simulink model "kurtosis"  (R2012b)
settings: Solver=ode45  StartTime=0.0  StopTime=3171  RelTol=1e-3
libraries: xbsIndex_r4 x3174, casper_library_flow_control x64, casper_library_misc x1, simulink_xsg_bridge x1
(part 6 of 24)

== system kurtosis/kurtosis/kurtosis_acc_bank_6/abs_x_4th_acc ==
  sync : Inport
  b : Inport  Port=2
  Convert : xbsIndex_r4/Convert  gui_display_data_type=Fixed-point  arith_type="Signed  (2's comp)"  n_bits=96  bin_pt=68  float_type=Single  exp_bits=8  fraction_bits=24  quantization=Truncate  overflow=Wrap  en=off  latency=0  dbl_ovrd=off  pipeline=off  block_type=convert
  DSP48E_0 : xbsIndex_r4/DSP48E  use_a=Direct from A Port  use_b=Direct from B Port  reset_preg=off  pattern_from_creg=on  pattern='000000000000'  mask_from_creg=on  pattern_mask='000000000000'  sel_rounding_mask=Select mask  use_op=off  use_creg=on  rst_all=off  en_all=off  use_pcin=off  use_carrycascin=off  use_multsignin=off  use_carryout=on  use_patterndetect=off  use_patternbdetect=off  use_overflow=off  use_underflow=off  use_acout=off  use_bcout=off  use_pcout=off  use_multsignout=off  use_carrycascout=off  pipeline_a=1  pipeline_b=1  pipeline_acout=1  pipeline_bcout=1  pipeline_c=on  pipeline_p=on  pipeline_mult=on  pipeline_opmode=on  pipeline_alumode=on  pipeline_carryin=on  pipeline_carryinsel=on  rst_a=off  rst_b=off  rst_c=off  rst_mult=off  rst_p=off  rst_carry_in=off  rst_alumode=off  rst_ctrl=off  en_a1=off  en_a2=off  en_b1=off  en_b2=off  en_c=off  en_mult=off  en_p=off  en_carry_in=off  en_alumode=off  en_multcarryin=off  en_ctrl=off  use_synth_model=off  addsub_mode=ONE48  xl_useadderonly=off  block_type=dsp48e
  DSP48E_1 : xbsIndex_r4/DSP48E  use_a=Direct from A Port  use_b=Direct from B Port  reset_preg=off  pattern_from_creg=on  pattern='000000000000'  mask_from_creg=on  pattern_mask='000000000000'  sel_rounding_mask=Select mask  use_op=off  use_creg=off  rst_all=off  en_all=off  use_pcin=off  use_carrycascin=off  use_multsignin=off  use_carryout=off  use_patterndetect=off  use_patternbdetect=off  use_overflow=off  use_underflow=off  use_acout=off  use_bcout=off  use_pcout=off  use_multsignout=off  use_carrycascout=off  pipeline_a=2  pipeline_b=2  pipeline_acout=1  pipeline_bcout=1  pipeline_c=on  pipeline_p=on  pipeline_mult=on  pipeline_opmode=on  pipeline_alumode=on  pipeline_carryin=off  pipeline_carryinsel=on  rst_a=off  rst_b=off  rst_c=off  rst_mult=off  rst_p=off  rst_carry_in=off  rst_alumode=off  rst_ctrl=off  en_a1=off  en_a2=off  en_b1=off  en_b2=off  en_c=off  en_mult=off  en_p=off  en_carry_in=off  en_alumode=off  en_multcarryin=off  en_ctrl=off  use_synth_model=off  addsub_mode=ONE48  xl_useadderonly=off  block_type=dsp48e
  DSP48_AB_splitter1 : Subsystem
  DSP48_AB_splitter2_sub : Subsystem
  Delay1 : xbsIndex_r4/Delay  rst=off  infoeditControl=Selection of Reset will increase slice count due to use of real FFs and instead of SRLs  en=off  latency=1  dbl_ovrd=off  reg_retiming=off  block_type=delay
  Mux : xbsIndex_r4/Mux  inputs=2  en=off  latency=0  precision=Full  arith_type=Unsigned  n_bits=16  bin_pt=14  quantization=Truncate  overflow=Wrap  dbl_ovrd=off  block_type=mux
  Mux1 : xbsIndex_r4/Mux  inputs=2  en=off  latency=0  precision=Full  arith_type=Unsigned  n_bits=16  bin_pt=14  quantization=Truncate  overflow=Wrap  dbl_ovrd=off  block_type=mux
  Register : xbsIndex_r4/Register  init=0  rst=off  en=off  dbl_ovrd=off  block_type=register
  Reinterpret : xbsIndex_r4/Reinterpret  force_arith_type=on  arith_type="Signed  (2's comp)"  force_bin_pt=on  bin_pt=0  block_type=reinterpret
  Reinterpret1 : xbsIndex_r4/Reinterpret  force_arith_type=on  arith_type="Signed  (2's comp)"  force_bin_pt=on  bin_pt=0  block_type=reinterpret
  Reinterpret2 : xbsIndex_r4/Reinterpret  force_arith_type=on  arith_type="Signed  (2's comp)"  force_bin_pt=on  bin_pt=68  block_type=reinterpret
  Slice : xbsIndex_r4/Slice  nbits=48  boolean_output=off  mode=Lower Bit Location + Width  bit1=0  base1=MSB of Input  bit0=0  base0=LSB of Input  dbl_ovrd=off  block_type=slice
  Slice2 : xbsIndex_r4/Slice  nbits=48  boolean_output=off  mode=Lower Bit Location + Width  bit1=0  base1=MSB of Input  bit0=48  base0=LSB of Input  dbl_ovrd=off  block_type=slice
  cram : Subsystem
  dsp48e_ctrl_init_xblock94 : Subsystem
  dsp48e_ctrl_init_xblock95 : Subsystem
  opmode_0_rst : xbsIndex_r4/Constant  const=12  gui_display_data_type=Fixed-point  arith_type=Unsigned  n_bits=7  bin_pt=0  preci_type=Single  exp_width=8  frac_width=24  explicit_period=on  period=1  equ=P=C  opselect=C  inp2=PCIN>>17  opr=+  inp1=P  carry=CIN  dbl_ovrd=off  block_type=constant
  opmode_1_rst : xbsIndex_r4/Constant  const=3  gui_display_data_type=Fixed-point  arith_type=Unsigned  n_bits=7  bin_pt=0  preci_type=Single  exp_width=8  frac_width=24  explicit_period=on  period=1  equ=P=C  opselect=C  inp2=PCIN>>17  opr=+  inp1=P  carry=CIN  dbl_ovrd=off  block_type=constant
  zero : xbsIndex_r4/Constant  const=0  gui_display_data_type=Fixed-point  arith_type=Signed (2's comp)  n_bits=48  bin_pt=0  preci_type=Single  exp_width=8  frac_width=24  explicit_period=on  period=1  equ=P=C  opselect=C  inp2=PCIN>>17  opr=+  inp1=P  carry=CIN  dbl_ovrd=off  block_type=constant
  +=b : Outport
  wires:
  sync/1 -> Mux1/1, Mux/1
  Reinterpret1/1 -> Slice2/1, Slice/1  "Reinterpret1_out1"
  dsp48e_ctrl_init_xblock95/4(carryinsel) -> DSP48E_1/6  "dsp48e_ctrl1_out4"
  dsp48e_ctrl_init_xblock95/2(alumode) -> DSP48E_1/4  "dsp48e_ctrl1_out2"
  dsp48e_ctrl_init_xblock95/1(opmode) -> Mux1/2  "dsp48e_ctrl1_out1"
  dsp48e_ctrl_init_xblock94/4(carryinsel) -> DSP48E_0/7  "dsp48e_ctrl0_out4"
  dsp48e_ctrl_init_xblock94/3(carryin) -> DSP48E_0/6  "dsp48e_ctrl0_out3"
  dsp48e_ctrl_init_xblock94/2(alumode) -> DSP48E_0/5  "dsp48e_ctrl0_out2"
  dsp48e_ctrl_init_xblock94/1(opmode) -> Mux/2  "dsp48e_ctrl0_out1"
  DSP48_AB_splitter2_sub/2(B) -> DSP48E_1/2  "DSP48_AB_splitter2_out2"
  DSP48_AB_splitter2_sub/1(A) -> DSP48E_1/1  "DSP48_AB_splitter2_out1"
  Slice2/1 -> DSP48_AB_splitter2_sub/1(A:B)  "Slice2_out1"
  zero/1 -> DSP48_AB_splitter1/1(A:B)  "zero_out1"
  opmode_1_rst/1 -> Mux1/3  "opmode_1_rst_out1"
  opmode_0_rst/1 -> Mux/3  "opmode_0_rst_out1"
  cram/1(Out) -> Reinterpret2/1  "cram_out1"
  Register/1 -> cram/2(In2)  "Register_out1"
  DSP48E_1/1 -> cram/1(In1)  "DSP48E_1_out1"
  Slice/1 -> Reinterpret/1  "Slice_out1"
  Reinterpret2/1 -> +=b/1
  Convert/1 -> Reinterpret1/1  "Convert_out1"
  Reinterpret/1 -> DSP48E_0/3  "Reinterpret_out1"
  DSP48E_0/1 -> Register/1  "DSP48E_0_out1"
  Mux1/1 -> Delay1/1  "Mux1_out1"
  Mux/1 -> DSP48E_0/4  "Mux_out1"
  Delay1/1 -> DSP48E_1/3  "Delay1_out1"
  DSP48_AB_splitter1/2(B) -> DSP48E_0/2  "DSP48_AB_splitter1_out2"
  DSP48_AB_splitter1/1(A) -> DSP48E_0/1  "DSP48_AB_splitter1_out1"
  DSP48E_0/2 -> DSP48E_1/5  "DSP48E_0_out2"
  b/1 -> Convert/1

== system kurtosis/kurtosis/kurtosis_acc_bank_6/abs_x_sq_acc ==
  sync : Inport
  b : Inport  Port=2
  Convert : xbsIndex_r4/Convert  gui_display_data_type=Fixed-point  arith_type="Signed  (2's comp)"  n_bits=96  bin_pt=34  float_type=Single  exp_bits=8  fraction_bits=24  quantization=Truncate  overflow=Wrap  en=off  latency=0  dbl_ovrd=off  pipeline=off  block_type=convert
  DSP48E_0 : xbsIndex_r4/DSP48E  use_a=Direct from A Port  use_b=Direct from B Port  reset_preg=off  pattern_from_creg=on  pattern='000000000000'  mask_from_creg=on  pattern_mask='000000000000'  sel_rounding_mask=Select mask  use_op=off  use_creg=on  rst_all=off  en_all=off  use_pcin=off  use_carrycascin=off  use_multsignin=off  use_carryout=on  use_patterndetect=off  use_patternbdetect=off  use_overflow=off  use_underflow=off  use_acout=off  use_bcout=off  use_pcout=off  use_multsignout=off  use_carrycascout=off  pipeline_a=1  pipeline_b=1  pipeline_acout=1  pipeline_bcout=1  pipeline_c=on  pipeline_p=on  pipeline_mult=on  pipeline_opmode=on  pipeline_alumode=on  pipeline_carryin=on  pipeline_carryinsel=on  rst_a=off  rst_b=off  rst_c=off  rst_mult=off  rst_p=off  rst_carry_in=off  rst_alumode=off  rst_ctrl=off  en_a1=off  en_a2=off  en_b1=off  en_b2=off  en_c=off  en_mult=off  en_p=off  en_carry_in=off  en_alumode=off  en_multcarryin=off  en_ctrl=off  use_synth_model=off  addsub_mode=ONE48  xl_useadderonly=off  block_type=dsp48e
  DSP48E_1 : xbsIndex_r4/DSP48E  use_a=Direct from A Port  use_b=Direct from B Port  reset_preg=off  pattern_from_creg=on  pattern='000000000000'  mask_from_creg=on  pattern_mask='000000000000'  sel_rounding_mask=Select mask  use_op=off  use_creg=off  rst_all=off  en_all=off  use_pcin=off  use_carrycascin=off  use_multsignin=off  use_carryout=off  use_patterndetect=off  use_patternbdetect=off  use_overflow=off  use_underflow=off  use_acout=off  use_bcout=off  use_pcout=off  use_multsignout=off  use_carrycascout=off  pipeline_a=2  pipeline_b=2  pipeline_acout=1  pipeline_bcout=1  pipeline_c=on  pipeline_p=on  pipeline_mult=on  pipeline_opmode=on  pipeline_alumode=on  pipeline_carryin=off  pipeline_carryinsel=on  rst_a=off  rst_b=off  rst_c=off  rst_mult=off  rst_p=off  rst_carry_in=off  rst_alumode=off  rst_ctrl=off  en_a1=off  en_a2=off  en_b1=off  en_b2=off  en_c=off  en_mult=off  en_p=off  en_carry_in=off  en_alumode=off  en_multcarryin=off  en_ctrl=off  use_synth_model=off  addsub_mode=ONE48  xl_useadderonly=off  block_type=dsp48e
  DSP48_AB_splitter1 : Subsystem
  DSP48_AB_splitter2_sub : Subsystem
  Delay1 : xbsIndex_r4/Delay  rst=off  infoeditControl=Selection of Reset will increase slice count due to use of real FFs and instead of SRLs  en=off  latency=1  dbl_ovrd=off  reg_retiming=off  block_type=delay
  Mux : xbsIndex_r4/Mux  inputs=2  en=off  latency=0  precision=Full  arith_type=Unsigned  n_bits=16  bin_pt=14  quantization=Truncate  overflow=Wrap  dbl_ovrd=off  block_type=mux
  Mux1 : xbsIndex_r4/Mux  inputs=2  en=off  latency=0  precision=Full  arith_type=Unsigned  n_bits=16  bin_pt=14  quantization=Truncate  overflow=Wrap  dbl_ovrd=off  block_type=mux
  Register : xbsIndex_r4/Register  init=0  rst=off  en=off  dbl_ovrd=off  block_type=register
  Reinterpret : xbsIndex_r4/Reinterpret  force_arith_type=on  arith_type="Signed  (2's comp)"  force_bin_pt=on  bin_pt=0  block_type=reinterpret
  Reinterpret1 : xbsIndex_r4/Reinterpret  force_arith_type=on  arith_type="Signed  (2's comp)"  force_bin_pt=on  bin_pt=0  block_type=reinterpret
  Reinterpret2 : xbsIndex_r4/Reinterpret  force_arith_type=on  arith_type="Signed  (2's comp)"  force_bin_pt=on  bin_pt=34  block_type=reinterpret
  Slice : xbsIndex_r4/Slice  nbits=48  boolean_output=off  mode=Lower Bit Location + Width  bit1=0  base1=MSB of Input  bit0=0  base0=LSB of Input  dbl_ovrd=off  block_type=slice
  Slice2 : xbsIndex_r4/Slice  nbits=48  boolean_output=off  mode=Lower Bit Location + Width  bit1=0  base1=MSB of Input  bit0=48  base0=LSB of Input  dbl_ovrd=off  block_type=slice
  cram : Subsystem
  dsp48e_ctrl_init_xblock92 : Subsystem
  dsp48e_ctrl_init_xblock93 : Subsystem
  opmode_0_rst : xbsIndex_r4/Constant  const=12  gui_display_data_type=Fixed-point  arith_type=Unsigned  n_bits=7  bin_pt=0  preci_type=Single  exp_width=8  frac_width=24  explicit_period=on  period=1  equ=P=C  opselect=C  inp2=PCIN>>17  opr=+  inp1=P  carry=CIN  dbl_ovrd=off  block_type=constant
  opmode_1_rst : xbsIndex_r4/Constant  const=3  gui_display_data_type=Fixed-point  arith_type=Unsigned  n_bits=7  bin_pt=0  preci_type=Single  exp_width=8  frac_width=24  explicit_period=on  period=1  equ=P=C  opselect=C  inp2=PCIN>>17  opr=+  inp1=P  carry=CIN  dbl_ovrd=off  block_type=constant
  zero : xbsIndex_r4/Constant  const=0  gui_display_data_type=Fixed-point  arith_type=Signed (2's comp)  n_bits=48  bin_pt=0  preci_type=Single  exp_width=8  frac_width=24  explicit_period=on  period=1  equ=P=C  opselect=C  inp2=PCIN>>17  opr=+  inp1=P  carry=CIN  dbl_ovrd=off  block_type=constant
  +=b : Outport
  wires:
  sync/1 -> Mux1/1, Mux/1
  Reinterpret1/1 -> Slice2/1, Slice/1  "Reinterpret1_out1"
  dsp48e_ctrl_init_xblock93/4(carryinsel) -> DSP48E_1/6  "dsp48e_ctrl1_out4"
  dsp48e_ctrl_init_xblock93/2(alumode) -> DSP48E_1/4  "dsp48e_ctrl1_out2"
  dsp48e_ctrl_init_xblock93/1(opmode) -> Mux1/2  "dsp48e_ctrl1_out1"
  dsp48e_ctrl_init_xblock92/4(carryinsel) -> DSP48E_0/7  "dsp48e_ctrl0_out4"
  dsp48e_ctrl_init_xblock92/3(carryin) -> DSP48E_0/6  "dsp48e_ctrl0_out3"
  dsp48e_ctrl_init_xblock92/2(alumode) -> DSP48E_0/5  "dsp48e_ctrl0_out2"
  dsp48e_ctrl_init_xblock92/1(opmode) -> Mux/2  "dsp48e_ctrl0_out1"
  DSP48_AB_splitter2_sub/2(B) -> DSP48E_1/2  "DSP48_AB_splitter2_out2"
  DSP48_AB_splitter2_sub/1(A) -> DSP48E_1/1  "DSP48_AB_splitter2_out1"
  Slice2/1 -> DSP48_AB_splitter2_sub/1(A:B)  "Slice2_out1"
  zero/1 -> DSP48_AB_splitter1/1(A:B)  "zero_out1"
  opmode_1_rst/1 -> Mux1/3  "opmode_1_rst_out1"
  opmode_0_rst/1 -> Mux/3  "opmode_0_rst_out1"
  cram/1(Out) -> Reinterpret2/1  "cram_out1"
  Register/1 -> cram/2(In2)  "Register_out1"
  DSP48E_1/1 -> cram/1(In1)  "DSP48E_1_out1"
  Slice/1 -> Reinterpret/1  "Slice_out1"
  Reinterpret2/1 -> +=b/1
  Convert/1 -> Reinterpret1/1  "Convert_out1"
  Reinterpret/1 -> DSP48E_0/3  "Reinterpret_out1"
  DSP48E_0/1 -> Register/1  "DSP48E_0_out1"
  Mux1/1 -> Delay1/1  "Mux1_out1"
  Mux/1 -> DSP48E_0/4  "Mux_out1"
  Delay1/1 -> DSP48E_1/3  "Delay1_out1"
  DSP48_AB_splitter1/2(B) -> DSP48E_0/2  "DSP48_AB_splitter1_out2"
  DSP48_AB_splitter1/1(A) -> DSP48E_0/1  "DSP48_AB_splitter1_out1"
  DSP48E_0/2 -> DSP48E_1/5  "DSP48E_0_out2"
  b/1 -> Convert/1

== system kurtosis/kurtosis/kurtosis_acc_bank_6/acc_rst ==
  sync : Inport
  Constant5 : xbsIndex_r4/Constant  const=1023  gui_display_data_type=Fixed-point  arith_type=Unsigned  n_bits=11  bin_pt=0  preci_type=Single  exp_width=8  frac_width=24  explicit_period=on  period=1  equ=P=C  opselect=C  inp2=PCIN>>17  opr=+  inp1=P  carry=CIN  dbl_ovrd=off  block_type=constant
  Counter : xbsIndex_r4/Counter  cnt_type=Free Running  cnt_to=Inf  operation=Up  start_count=0  cnt_by_val=1  arith_type=Unsigned  n_bits=10  bin_pt=0  load_pin=off  rst=on  en=off  explicit_period=on  period=1  dbl_ovrd=off  use_behavioral_HDL=off  implementation=Fabric  block_type=counter
  Logical : xbsIndex_r4/Logical  logical_function=OR  inputs=2  en=off  latency=0  precision=Full  arith_type=Unsigned  n_bits=16  bin_pt=0  align_bp=on  dbl_ovrd=off  block_type=logical
  Relational : xbsIndex_r4/Relational  mode=a=b  en=off  latency=0  dbl_ovrd=off  block_type=relational
  acc_del : xbsIndex_r4/Delay  rst=off  infoeditControl=Selection of Reset will increase slice count due to use of real FFs and instead of SRLs  en=off  latency=2  dbl_ovrd=off  reg_retiming=off  block_type=delay
  sync_del : xbsIndex_r4/Delay  rst=off  infoeditControl=Selection of Reset will increase slice count due to use of real FFs and instead of SRLs  en=off  latency=1  dbl_ovrd=off  reg_retiming=off  block_type=delay
  acc_rst : Outport
  sync_out : Outport  Port=2
  wires:
  sync/1 -> Logical/2, Counter/1
  Relational/1 -> sync_del/1, acc_del/1  "Relational_out1"
  sync_del/1 -> Logical/1  "sync_del_out1"
  acc_del/1 -> sync_out/1
  Constant5/1 -> Relational/2  "Constant5_out1"
  Counter/1 -> Relational/1  "Counter_out1"
  Logical/1 -> acc_rst/1

== system kurtosis/kurtosis/kurtosis_acc_bank_6/x_acc ==
  sync : Inport
  x : Inport  Port=2
  c_to_ri : Subsystem
  im_acc : Subsystem
  re_acc : Subsystem
  x_re_acc : Outport
  x_im_acc : Outport  Port=2
  wires:
  sync/1 -> im_acc/1(sync), re_acc/1(sync)
  im_acc/1(+=b) -> x_im_acc/1
  c_to_ri/2(im) -> im_acc/2(b)  "x_im"
  re_acc/1(+=b) -> x_re_acc/1
  c_to_ri/1(re) -> re_acc/2(b)  "x_re"
  x/1 -> c_to_ri/1(c)

== system kurtosis/kurtosis/kurtosis_acc_bank_6/x_cube_acc ==
  sync : Inport
  x : Inport  Port=2
  c_to_ri : Subsystem
  im_acc : Subsystem
  re_acc : Subsystem
  x_re_acc : Outport
  x_im_acc : Outport  Port=2
  wires:
  sync/1 -> im_acc/1(sync), re_acc/1(sync)
  im_acc/1(+=b) -> x_im_acc/1
  c_to_ri/2(im) -> im_acc/2(b)  "x_im"
  re_acc/1(+=b) -> x_re_acc/1
  c_to_ri/1(re) -> re_acc/2(b)  "x_re"
  x/1 -> c_to_ri/1(c)

== system kurtosis/kurtosis/kurtosis_acc_bank_6/x_sq_acc ==
  sync : Inport
  x : Inport  Port=2
  c_to_ri : Subsystem
  im_acc : Subsystem
  re_acc : Subsystem
  x_re_acc : Outport
  x_im_acc : Outport  Port=2
  wires:
  sync/1 -> im_acc/1(sync), re_acc/1(sync)
  im_acc/1(+=b) -> x_im_acc/1
  c_to_ri/2(im) -> im_acc/2(b)  "x_im"
  re_acc/1(+=b) -> x_re_acc/1
  c_to_ri/1(re) -> re_acc/2(b)  "x_re"
  x/1 -> c_to_ri/1(c)

== system kurtosis/kurtosis/kurtosis_acc_bank_7/abs_x_4th_acc ==
  sync : Inport
  b : Inport  Port=2
  Convert : xbsIndex_r4/Convert  gui_display_data_type=Fixed-point  arith_type="Signed  (2's comp)"  n_bits=96  bin_pt=68  float_type=Single  exp_bits=8  fraction_bits=24  quantization=Truncate  overflow=Wrap  en=off  latency=0  dbl_ovrd=off  pipeline=off  block_type=convert
  DSP48E_0 : xbsIndex_r4/DSP48E  use_a=Direct from A Port  use_b=Direct from B Port  reset_preg=off  pattern_from_creg=on  pattern='000000000000'  mask_from_creg=on  pattern_mask='000000000000'  sel_rounding_mask=Select mask  use_op=off  use_creg=on  rst_all=off  en_all=off  use_pcin=off  use_carrycascin=off  use_multsignin=off  use_carryout=on  use_patterndetect=off  use_patternbdetect=off  use_overflow=off  use_underflow=off  use_acout=off  use_bcout=off  use_pcout=off  use_multsignout=off  use_carrycascout=off  pipeline_a=1  pipeline_b=1  pipeline_acout=1  pipeline_bcout=1  pipeline_c=on  pipeline_p=on  pipeline_mult=on  pipeline_opmode=on  pipeline_alumode=on  pipeline_carryin=on  pipeline_carryinsel=on  rst_a=off  rst_b=off  rst_c=off  rst_mult=off  rst_p=off  rst_carry_in=off  rst_alumode=off  rst_ctrl=off  en_a1=off  en_a2=off  en_b1=off  en_b2=off  en_c=off  en_mult=off  en_p=off  en_carry_in=off  en_alumode=off  en_multcarryin=off  en_ctrl=off  use_synth_model=off  addsub_mode=ONE48  xl_useadderonly=off  block_type=dsp48e
  DSP48E_1 : xbsIndex_r4/DSP48E  use_a=Direct from A Port  use_b=Direct from B Port  reset_preg=off  pattern_from_creg=on  pattern='000000000000'  mask_from_creg=on  pattern_mask='000000000000'  sel_rounding_mask=Select mask  use_op=off  use_creg=off  rst_all=off  en_all=off  use_pcin=off  use_carrycascin=off  use_multsignin=off  use_carryout=off  use_patterndetect=off  use_patternbdetect=off  use_overflow=off  use_underflow=off  use_acout=off  use_bcout=off  use_pcout=off  use_multsignout=off  use_carrycascout=off  pipeline_a=2  pipeline_b=2  pipeline_acout=1  pipeline_bcout=1  pipeline_c=on  pipeline_p=on  pipeline_mult=on  pipeline_opmode=on  pipeline_alumode=on  pipeline_carryin=off  pipeline_carryinsel=on  rst_a=off  rst_b=off  rst_c=off  rst_mult=off  rst_p=off  rst_carry_in=off  rst_alumode=off  rst_ctrl=off  en_a1=off  en_a2=off  en_b1=off  en_b2=off  en_c=off  en_mult=off  en_p=off  en_carry_in=off  en_alumode=off  en_multcarryin=off  en_ctrl=off  use_synth_model=off  addsub_mode=ONE48  xl_useadderonly=off  block_type=dsp48e
  DSP48_AB_splitter1 : Subsystem
  DSP48_AB_splitter2_sub : Subsystem
  Delay1 : xbsIndex_r4/Delay  rst=off  infoeditControl=Selection of Reset will increase slice count due to use of real FFs and instead of SRLs  en=off  latency=1  dbl_ovrd=off  reg_retiming=off  block_type=delay
  Mux : xbsIndex_r4/Mux  inputs=2  en=off  latency=0  precision=Full  arith_type=Unsigned  n_bits=16  bin_pt=14  quantization=Truncate  overflow=Wrap  dbl_ovrd=off  block_type=mux
  Mux1 : xbsIndex_r4/Mux  inputs=2  en=off  latency=0  precision=Full  arith_type=Unsigned  n_bits=16  bin_pt=14  quantization=Truncate  overflow=Wrap  dbl_ovrd=off  block_type=mux
  Register : xbsIndex_r4/Register  init=0  rst=off  en=off  dbl_ovrd=off  block_type=register
  Reinterpret : xbsIndex_r4/Reinterpret  force_arith_type=on  arith_type="Signed  (2's comp)"  force_bin_pt=on  bin_pt=0  block_type=reinterpret
  Reinterpret1 : xbsIndex_r4/Reinterpret  force_arith_type=on  arith_type="Signed  (2's comp)"  force_bin_pt=on  bin_pt=0  block_type=reinterpret
  Reinterpret2 : xbsIndex_r4/Reinterpret  force_arith_type=on  arith_type="Signed  (2's comp)"  force_bin_pt=on  bin_pt=68  block_type=reinterpret
  Slice : xbsIndex_r4/Slice  nbits=48  boolean_output=off  mode=Lower Bit Location + Width  bit1=0  base1=MSB of Input  bit0=0  base0=LSB of Input  dbl_ovrd=off  block_type=slice
  Slice2 : xbsIndex_r4/Slice  nbits=48  boolean_output=off  mode=Lower Bit Location + Width  bit1=0  base1=MSB of Input  bit0=48  base0=LSB of Input  dbl_ovrd=off  block_type=slice
  cram : Subsystem
  dsp48e_ctrl_init_xblock110 : Subsystem
  dsp48e_ctrl_init_xblock111 : Subsystem
  opmode_0_rst : xbsIndex_r4/Constant  const=12  gui_display_data_type=Fixed-point  arith_type=Unsigned  n_bits=7  bin_pt=0  preci_type=Single  exp_width=8  frac_width=24  explicit_period=on  period=1  equ=P=C  opselect=C  inp2=PCIN>>17  opr=+  inp1=P  carry=CIN  dbl_ovrd=off  block_type=constant
  opmode_1_rst : xbsIndex_r4/Constant  const=3  gui_display_data_type=Fixed-point  arith_type=Unsigned  n_bits=7  bin_pt=0  preci_type=Single  exp_width=8  frac_width=24  explicit_period=on  period=1  equ=P=C  opselect=C  inp2=PCIN>>17  opr=+  inp1=P  carry=CIN  dbl_ovrd=off  block_type=constant
  zero : xbsIndex_r4/Constant  const=0  gui_display_data_type=Fixed-point  arith_type=Signed (2's comp)  n_bits=48  bin_pt=0  preci_type=Single  exp_width=8  frac_width=24  explicit_period=on  period=1  equ=P=C  opselect=C  inp2=PCIN>>17  opr=+  inp1=P  carry=CIN  dbl_ovrd=off  block_type=constant
  +=b : Outport
  wires:
  sync/1 -> Mux1/1, Mux/1
  Reinterpret1/1 -> Slice2/1, Slice/1  "Reinterpret1_out1"
  dsp48e_ctrl_init_xblock111/4(carryinsel) -> DSP48E_1/6  "dsp48e_ctrl1_out4"
  dsp48e_ctrl_init_xblock111/2(alumode) -> DSP48E_1/4  "dsp48e_ctrl1_out2"
  dsp48e_ctrl_init_xblock111/1(opmode) -> Mux1/2  "dsp48e_ctrl1_out1"
  dsp48e_ctrl_init_xblock110/4(carryinsel) -> DSP48E_0/7  "dsp48e_ctrl0_out4"
  dsp48e_ctrl_init_xblock110/3(carryin) -> DSP48E_0/6  "dsp48e_ctrl0_out3"
  dsp48e_ctrl_init_xblock110/2(alumode) -> DSP48E_0/5  "dsp48e_ctrl0_out2"
  dsp48e_ctrl_init_xblock110/1(opmode) -> Mux/2  "dsp48e_ctrl0_out1"
  DSP48_AB_splitter2_sub/2(B) -> DSP48E_1/2  "DSP48_AB_splitter2_out2"
  DSP48_AB_splitter2_sub/1(A) -> DSP48E_1/1  "DSP48_AB_splitter2_out1"
  Slice2/1 -> DSP48_AB_splitter2_sub/1(A:B)  "Slice2_out1"
  zero/1 -> DSP48_AB_splitter1/1(A:B)  "zero_out1"
  opmode_1_rst/1 -> Mux1/3  "opmode_1_rst_out1"
  opmode_0_rst/1 -> Mux/3  "opmode_0_rst_out1"
  cram/1(Out) -> Reinterpret2/1  "cram_out1"
  Register/1 -> cram/2(In2)  "Register_out1"
  DSP48E_1/1 -> cram/1(In1)  "DSP48E_1_out1"
  Slice/1 -> Reinterpret/1  "Slice_out1"
  Reinterpret2/1 -> +=b/1
  Convert/1 -> Reinterpret1/1  "Convert_out1"
  Reinterpret/1 -> DSP48E_0/3  "Reinterpret_out1"
  DSP48E_0/1 -> Register/1  "DSP48E_0_out1"
  Mux1/1 -> Delay1/1  "Mux1_out1"
  Mux/1 -> DSP48E_0/4  "Mux_out1"
  Delay1/1 -> DSP48E_1/3  "Delay1_out1"
  DSP48_AB_splitter1/2(B) -> DSP48E_0/2  "DSP48_AB_splitter1_out2"
  DSP48_AB_splitter1/1(A) -> DSP48E_0/1  "DSP48_AB_splitter1_out1"
  DSP48E_0/2 -> DSP48E_1/5  "DSP48E_0_out2"
  b/1 -> Convert/1

== system kurtosis/kurtosis/kurtosis_acc_bank_7/abs_x_sq_acc ==
  sync : Inport
  b : Inport  Port=2
  Convert : xbsIndex_r4/Convert  gui_display_data_type=Fixed-point  arith_type="Signed  (2's comp)"  n_bits=96  bin_pt=34  float_type=Single  exp_bits=8  fraction_bits=24  quantization=Truncate  overflow=Wrap  en=off  latency=0  dbl_ovrd=off  pipeline=off  block_type=convert
  DSP48E_0 : xbsIndex_r4/DSP48E  use_a=Direct from A Port  use_b=Direct from B Port  reset_preg=off  pattern_from_creg=on  pattern='000000000000'  mask_from_creg=on  pattern_mask='000000000000'  sel_rounding_mask=Select mask  use_op=off  use_creg=on  rst_all=off  en_all=off  use_pcin=off  use_carrycascin=off  use_multsignin=off  use_carryout=on  use_patterndetect=off  use_patternbdetect=off  use_overflow=off  use_underflow=off  use_acout=off  use_bcout=off  use_pcout=off  use_multsignout=off  use_carrycascout=off  pipeline_a=1  pipeline_b=1  pipeline_acout=1  pipeline_bcout=1  pipeline_c=on  pipeline_p=on  pipeline_mult=on  pipeline_opmode=on  pipeline_alumode=on  pipeline_carryin=on  pipeline_carryinsel=on  rst_a=off  rst_b=off  rst_c=off  rst_mult=off  rst_p=off  rst_carry_in=off  rst_alumode=off  rst_ctrl=off  en_a1=off  en_a2=off  en_b1=off  en_b2=off  en_c=off  en_mult=off  en_p=off  en_carry_in=off  en_alumode=off  en_multcarryin=off  en_ctrl=off  use_synth_model=off  addsub_mode=ONE48  xl_useadderonly=off  block_type=dsp48e
  DSP48E_1 : xbsIndex_r4/DSP48E  use_a=Direct from A Port  use_b=Direct from B Port  reset_preg=off  pattern_from_creg=on  pattern='000000000000'  mask_from_creg=on  pattern_mask='000000000000'  sel_rounding_mask=Select mask  use_op=off  use_creg=off  rst_all=off  en_all=off  use_pcin=off  use_carrycascin=off  use_multsignin=off  use_carryout=off  use_patterndetect=off  use_patternbdetect=off  use_overflow=off  use_underflow=off  use_acout=off  use_bcout=off  use_pcout=off  use_multsignout=off  use_carrycascout=off  pipeline_a=2  pipeline_b=2  pipeline_acout=1  pipeline_bcout=1  pipeline_c=on  pipeline_p=on  pipeline_mult=on  pipeline_opmode=on  pipeline_alumode=on  pipeline_carryin=off  pipeline_carryinsel=on  rst_a=off  rst_b=off  rst_c=off  rst_mult=off  rst_p=off  rst_carry_in=off  rst_alumode=off  rst_ctrl=off  en_a1=off  en_a2=off  en_b1=off  en_b2=off  en_c=off  en_mult=off  en_p=off  en_carry_in=off  en_alumode=off  en_multcarryin=off  en_ctrl=off  use_synth_model=off  addsub_mode=ONE48  xl_useadderonly=off  block_type=dsp48e
  DSP48_AB_splitter1 : Subsystem
  DSP48_AB_splitter2_sub : Subsystem
  Delay1 : xbsIndex_r4/Delay  rst=off  infoeditControl=Selection of Reset will increase slice count due to use of real FFs and instead of SRLs  en=off  latency=1  dbl_ovrd=off  reg_retiming=off  block_type=delay
  Mux : xbsIndex_r4/Mux  inputs=2  en=off  latency=0  precision=Full  arith_type=Unsigned  n_bits=16  bin_pt=14  quantization=Truncate  overflow=Wrap  dbl_ovrd=off  block_type=mux
  Mux1 : xbsIndex_r4/Mux  inputs=2  en=off  latency=0  precision=Full  arith_type=Unsigned  n_bits=16  bin_pt=14  quantization=Truncate  overflow=Wrap  dbl_ovrd=off  block_type=mux
  Register : xbsIndex_r4/Register  init=0  rst=off  en=off  dbl_ovrd=off  block_type=register
  Reinterpret : xbsIndex_r4/Reinterpret  force_arith_type=on  arith_type="Signed  (2's comp)"  force_bin_pt=on  bin_pt=0  block_type=reinterpret
  Reinterpret1 : xbsIndex_r4/Reinterpret  force_arith_type=on  arith_type="Signed  (2's comp)"  force_bin_pt=on  bin_pt=0  block_type=reinterpret
  Reinterpret2 : xbsIndex_r4/Reinterpret  force_arith_type=on  arith_type="Signed  (2's comp)"  force_bin_pt=on  bin_pt=34  block_type=reinterpret
  Slice : xbsIndex_r4/Slice  nbits=48  boolean_output=off  mode=Lower Bit Location + Width  bit1=0  base1=MSB of Input  bit0=0  base0=LSB of Input  dbl_ovrd=off  block_type=slice
  Slice2 : xbsIndex_r4/Slice  nbits=48  boolean_output=off  mode=Lower Bit Location + Width  bit1=0  base1=MSB of Input  bit0=48  base0=LSB of Input  dbl_ovrd=off  block_type=slice
  cram : Subsystem
  dsp48e_ctrl_init_xblock108 : Subsystem
  dsp48e_ctrl_init_xblock109 : Subsystem
  opmode_0_rst : xbsIndex_r4/Constant  const=12  gui_display_data_type=Fixed-point  arith_type=Unsigned  n_bits=7  bin_pt=0  preci_type=Single  exp_width=8  frac_width=24  explicit_period=on  period=1  equ=P=C  opselect=C  inp2=PCIN>>17  opr=+  inp1=P  carry=CIN  dbl_ovrd=off  block_type=constant
  opmode_1_rst : xbsIndex_r4/Constant  const=3  gui_display_data_type=Fixed-point  arith_type=Unsigned  n_bits=7  bin_pt=0  preci_type=Single  exp_width=8  frac_width=24  explicit_period=on  period=1  equ=P=C  opselect=C  inp2=PCIN>>17  opr=+  inp1=P  carry=CIN  dbl_ovrd=off  block_type=constant
  zero : xbsIndex_r4/Constant  const=0  gui_display_data_type=Fixed-point  arith_type=Signed (2's comp)  n_bits=48  bin_pt=0  preci_type=Single  exp_width=8  frac_width=24  explicit_period=on  period=1  equ=P=C  opselect=C  inp2=PCIN>>17  opr=+  inp1=P  carry=CIN  dbl_ovrd=off  block_type=constant
  +=b : Outport
  wires:
  sync/1 -> Mux1/1, Mux/1
  Reinterpret1/1 -> Slice2/1, Slice/1  "Reinterpret1_out1"
  dsp48e_ctrl_init_xblock109/4(carryinsel) -> DSP48E_1/6  "dsp48e_ctrl1_out4"
  dsp48e_ctrl_init_xblock109/2(alumode) -> DSP48E_1/4  "dsp48e_ctrl1_out2"
  dsp48e_ctrl_init_xblock109/1(opmode) -> Mux1/2  "dsp48e_ctrl1_out1"
  dsp48e_ctrl_init_xblock108/4(carryinsel) -> DSP48E_0/7  "dsp48e_ctrl0_out4"
  dsp48e_ctrl_init_xblock108/3(carryin) -> DSP48E_0/6  "dsp48e_ctrl0_out3"
  dsp48e_ctrl_init_xblock108/2(alumode) -> DSP48E_0/5  "dsp48e_ctrl0_out2"
  dsp48e_ctrl_init_xblock108/1(opmode) -> Mux/2  "dsp48e_ctrl0_out1"
  DSP48_AB_splitter2_sub/2(B) -> DSP48E_1/2  "DSP48_AB_splitter2_out2"
  DSP48_AB_splitter2_sub/1(A) -> DSP48E_1/1  "DSP48_AB_splitter2_out1"
  Slice2/1 -> DSP48_AB_splitter2_sub/1(A:B)  "Slice2_out1"
  zero/1 -> DSP48_AB_splitter1/1(A:B)  "zero_out1"
  opmode_1_rst/1 -> Mux1/3  "opmode_1_rst_out1"
  opmode_0_rst/1 -> Mux/3  "opmode_0_rst_out1"
  cram/1(Out) -> Reinterpret2/1  "cram_out1"
  Register/1 -> cram/2(In2)  "Register_out1"
  DSP48E_1/1 -> cram/1(In1)  "DSP48E_1_out1"
  Slice/1 -> Reinterpret/1  "Slice_out1"
  Reinterpret2/1 -> +=b/1
  Convert/1 -> Reinterpret1/1  "Convert_out1"
  Reinterpret/1 -> DSP48E_0/3  "Reinterpret_out1"
  DSP48E_0/1 -> Register/1  "DSP48E_0_out1"
  Mux1/1 -> Delay1/1  "Mux1_out1"
  Mux/1 -> DSP48E_0/4  "Mux_out1"
  Delay1/1 -> DSP48E_1/3  "Delay1_out1"
  DSP48_AB_splitter1/2(B) -> DSP48E_0/2  "DSP48_AB_splitter1_out2"
  DSP48_AB_splitter1/1(A) -> DSP48E_0/1  "DSP48_AB_splitter1_out1"
  DSP48E_0/2 -> DSP48E_1/5  "DSP48E_0_out2"
  b/1 -> Convert/1

== system kurtosis/kurtosis/kurtosis_acc_bank_7/acc_rst ==
  sync : Inport
  Constant5 : xbsIndex_r4/Constant  const=1023  gui_display_data_type=Fixed-point  arith_type=Unsigned  n_bits=11  bin_pt=0  preci_type=Single  exp_width=8  frac_width=24  explicit_period=on  period=1  equ=P=C  opselect=C  inp2=PCIN>>17  opr=+  inp1=P  carry=CIN  dbl_ovrd=off  block_type=constant
  Counter : xbsIndex_r4/Counter  cnt_type=Free Running  cnt_to=Inf  operation=Up  start_count=0  cnt_by_val=1  arith_type=Unsigned  n_bits=10  bin_pt=0  load_pin=off  rst=on  en=off  explicit_period=on  period=1  dbl_ovrd=off  use_behavioral_HDL=off  implementation=Fabric  block_type=counter
  Logical : xbsIndex_r4/Logical  logical_function=OR  inputs=2  en=off  latency=0  precision=Full  arith_type=Unsigned  n_bits=16  bin_pt=0  align_bp=on  dbl_ovrd=off  block_type=logical
  Relational : xbsIndex_r4/Relational  mode=a=b  en=off  latency=0  dbl_ovrd=off  block_type=relational
  acc_del : xbsIndex_r4/Delay  rst=off  infoeditControl=Selection of Reset will increase slice count due to use of real FFs and instead of SRLs  en=off  latency=2  dbl_ovrd=off  reg_retiming=off  block_type=delay
  sync_del : xbsIndex_r4/Delay  rst=off  infoeditControl=Selection of Reset will increase slice count due to use of real FFs and instead of SRLs  en=off  latency=1  dbl_ovrd=off  reg_retiming=off  block_type=delay
  acc_rst : Outport
  sync_out : Outport  Port=2
  wires:
  sync/1 -> Logical/2, Counter/1
  Relational/1 -> sync_del/1, acc_del/1  "Relational_out1"
  sync_del/1 -> Logical/1  "sync_del_out1"
  acc_del/1 -> sync_out/1
  Constant5/1 -> Relational/2  "Constant5_out1"
  Counter/1 -> Relational/1  "Counter_out1"
  Logical/1 -> acc_rst/1

== system kurtosis/kurtosis/kurtosis_acc_bank_7/x_acc ==
  sync : Inport
  x : Inport  Port=2
  c_to_ri : Subsystem
  im_acc : Subsystem
  re_acc : Subsystem
  x_re_acc : Outport
  x_im_acc : Outport  Port=2
  wires:
  sync/1 -> im_acc/1(sync), re_acc/1(sync)
  im_acc/1(+=b) -> x_im_acc/1
  c_to_ri/2(im) -> im_acc/2(b)  "x_im"
  re_acc/1(+=b) -> x_re_acc/1
  c_to_ri/1(re) -> re_acc/2(b)  "x_re"
  x/1 -> c_to_ri/1(c)

== system kurtosis/kurtosis/kurtosis_acc_bank_7/x_cube_acc ==
  sync : Inport
  x : Inport  Port=2
  c_to_ri : Subsystem
  im_acc : Subsystem
  re_acc : Subsystem
  x_re_acc : Outport
  x_im_acc : Outport  Port=2
  wires:
  sync/1 -> im_acc/1(sync), re_acc/1(sync)
  im_acc/1(+=b) -> x_im_acc/1
  c_to_ri/2(im) -> im_acc/2(b)  "x_im"
  re_acc/1(+=b) -> x_re_acc/1
  c_to_ri/1(re) -> re_acc/2(b)  "x_re"
  x/1 -> c_to_ri/1(c)

== system kurtosis/kurtosis/kurtosis_acc_bank_7/x_sq_acc ==
  sync : Inport
  x : Inport  Port=2
  c_to_ri : Subsystem
  im_acc : Subsystem
  re_acc : Subsystem
  x_re_acc : Outport
  x_im_acc : Outport  Port=2
  wires:
  sync/1 -> im_acc/1(sync), re_acc/1(sync)
  im_acc/1(+=b) -> x_im_acc/1
  c_to_ri/2(im) -> im_acc/2(b)  "x_im"
  re_acc/1(+=b) -> x_re_acc/1
  c_to_ri/1(re) -> re_acc/2(b)  "x_re"
  x/1 -> c_to_ri/1(c)

== system kurtosis/kurtosis/kurtosis_acc_bank_8/abs_x_4th_acc ==
  sync : Inport
  b : Inport  Port=2
  Convert : xbsIndex_r4/Convert  gui_display_data_type=Fixed-point  arith_type="Signed  (2's comp)"  n_bits=96  bin_pt=68  float_type=Single  exp_bits=8  fraction_bits=24  quantization=Truncate  overflow=Wrap  en=off  latency=0  dbl_ovrd=off  pipeline=off  block_type=convert
  DSP48E_0 : xbsIndex_r4/DSP48E  use_a=Direct from A Port  use_b=Direct from B Port  reset_preg=off  pattern_from_creg=on  pattern='000000000000'  mask_from_creg=on  pattern_mask='000000000000'  sel_rounding_mask=Select mask  use_op=off  use_creg=on  rst_all=off  en_all=off  use_pcin=off  use_carrycascin=off  use_multsignin=off  use_carryout=on  use_patterndetect=off  use_patternbdetect=off  use_overflow=off  use_underflow=off  use_acout=off  use_bcout=off  use_pcout=off  use_multsignout=off  use_carrycascout=off  pipeline_a=1  pipeline_b=1  pipeline_acout=1  pipeline_bcout=1  pipeline_c=on  pipeline_p=on  pipeline_mult=on  pipeline_opmode=on  pipeline_alumode=on  pipeline_carryin=on  pipeline_carryinsel=on  rst_a=off  rst_b=off  rst_c=off  rst_mult=off  rst_p=off  rst_carry_in=off  rst_alumode=off  rst_ctrl=off  en_a1=off  en_a2=off  en_b1=off  en_b2=off  en_c=off  en_mult=off  en_p=off  en_carry_in=off  en_alumode=off  en_multcarryin=off  en_ctrl=off  use_synth_model=off  addsub_mode=ONE48  xl_useadderonly=off  block_type=dsp48e
  DSP48E_1 : xbsIndex_r4/DSP48E  use_a=Direct from A Port  use_b=Direct from B Port  reset_preg=off  pattern_from_creg=on  pattern='000000000000'  mask_from_creg=on  pattern_mask='000000000000'  sel_rounding_mask=Select mask  use_op=off  use_creg=off  rst_all=off  en_all=off  use_pcin=off  use_carrycascin=off  use_multsignin=off  use_carryout=off  use_patterndetect=off  use_patternbdetect=off  use_overflow=off  use_underflow=off  use_acout=off  use_bcout=off  use_pcout=off  use_multsignout=off  use_carrycascout=off  pipeline_a=2  pipeline_b=2  pipeline_acout=1  pipeline_bcout=1  pipeline_c=on  pipeline_p=on  pipeline_mult=on  pipeline_opmode=on  pipeline_alumode=on  pipeline_carryin=off  pipeline_carryinsel=on  rst_a=off  rst_b=off  rst_c=off  rst_mult=off  rst_p=off  rst_carry_in=off  rst_alumode=off  rst_ctrl=off  en_a1=off  en_a2=off  en_b1=off  en_b2=off  en_c=off  en_mult=off  en_p=off  en_carry_in=off  en_alumode=off  en_multcarryin=off  en_ctrl=off  use_synth_model=off  addsub_mode=ONE48  xl_useadderonly=off  block_type=dsp48e
  DSP48_AB_splitter1 : Subsystem
  DSP48_AB_splitter2_sub : Subsystem
  Delay1 : xbsIndex_r4/Delay  rst=off  infoeditControl=Selection of Reset will increase slice count due to use of real FFs and instead of SRLs  en=off  latency=1  dbl_ovrd=off  reg_retiming=off  block_type=delay
  Mux : xbsIndex_r4/Mux  inputs=2  en=off  latency=0  precision=Full  arith_type=Unsigned  n_bits=16  bin_pt=14  quantization=Truncate  overflow=Wrap  dbl_ovrd=off  block_type=mux
  Mux1 : xbsIndex_r4/Mux  inputs=2  en=off  latency=0  precision=Full  arith_type=Unsigned  n_bits=16  bin_pt=14  quantization=Truncate  overflow=Wrap  dbl_ovrd=off  block_type=mux
  Register : xbsIndex_r4/Register  init=0  rst=off  en=off  dbl_ovrd=off  block_type=register
  Reinterpret : xbsIndex_r4/Reinterpret  force_arith_type=on  arith_type="Signed  (2's comp)"  force_bin_pt=on  bin_pt=0  block_type=reinterpret
  Reinterpret1 : xbsIndex_r4/Reinterpret  force_arith_type=on  arith_type="Signed  (2's comp)"  force_bin_pt=on  bin_pt=0  block_type=reinterpret
  Reinterpret2 : xbsIndex_r4/Reinterpret  force_arith_type=on  arith_type="Signed  (2's comp)"  force_bin_pt=on  bin_pt=68  block_type=reinterpret
  Slice : xbsIndex_r4/Slice  nbits=48  boolean_output=off  mode=Lower Bit Location + Width  bit1=0  base1=MSB of Input  bit0=0  base0=LSB of Input  dbl_ovrd=off  block_type=slice
  Slice2 : xbsIndex_r4/Slice  nbits=48  boolean_output=off  mode=Lower Bit Location + Width  bit1=0  base1=MSB of Input  bit0=48  base0=LSB of Input  dbl_ovrd=off  block_type=slice
  cram : Subsystem
  dsp48e_ctrl_init_xblock126 : Subsystem
  dsp48e_ctrl_init_xblock127 : Subsystem
  opmode_0_rst : xbsIndex_r4/Constant  const=12  gui_display_data_type=Fixed-point  arith_type=Unsigned  n_bits=7  bin_pt=0  preci_type=Single  exp_width=8  frac_width=24  explicit_period=on  period=1  equ=P=C  opselect=C  inp2=PCIN>>17  opr=+  inp1=P  carry=CIN  dbl_ovrd=off  block_type=constant
  opmode_1_rst : xbsIndex_r4/Constant  const=3  gui_display_data_type=Fixed-point  arith_type=Unsigned  n_bits=7  bin_pt=0  preci_type=Single  exp_width=8  frac_width=24  explicit_period=on  period=1  equ=P=C  opselect=C  inp2=PCIN>>17  opr=+  inp1=P  carry=CIN  dbl_ovrd=off  block_type=constant
  zero : xbsIndex_r4/Constant  const=0  gui_display_data_type=Fixed-point  arith_type=Signed (2's comp)  n_bits=48  bin_pt=0  preci_type=Single  exp_width=8  frac_width=24  explicit_period=on  period=1  equ=P=C  opselect=C  inp2=PCIN>>17  opr=+  inp1=P  carry=CIN  dbl_ovrd=off  block_type=constant
  +=b : Outport
  wires:
  sync/1 -> Mux1/1, Mux/1
  Reinterpret1/1 -> Slice2/1, Slice/1  "Reinterpret1_out1"
  dsp48e_ctrl_init_xblock127/4(carryinsel) -> DSP48E_1/6  "dsp48e_ctrl1_out4"
  dsp48e_ctrl_init_xblock127/2(alumode) -> DSP48E_1/4  "dsp48e_ctrl1_out2"
  dsp48e_ctrl_init_xblock127/1(opmode) -> Mux1/2  "dsp48e_ctrl1_out1"
  dsp48e_ctrl_init_xblock126/4(carryinsel) -> DSP48E_0/7  "dsp48e_ctrl0_out4"
  dsp48e_ctrl_init_xblock126/3(carryin) -> DSP48E_0/6  "dsp48e_ctrl0_out3"
  dsp48e_ctrl_init_xblock126/2(alumode) -> DSP48E_0/5  "dsp48e_ctrl0_out2"
  dsp48e_ctrl_init_xblock126/1(opmode) -> Mux/2  "dsp48e_ctrl0_out1"
  DSP48_AB_splitter2_sub/2(B) -> DSP48E_1/2  "DSP48_AB_splitter2_out2"
  DSP48_AB_splitter2_sub/1(A) -> DSP48E_1/1  "DSP48_AB_splitter2_out1"
  Slice2/1 -> DSP48_AB_splitter2_sub/1(A:B)  "Slice2_out1"
  zero/1 -> DSP48_AB_splitter1/1(A:B)  "zero_out1"
  opmode_1_rst/1 -> Mux1/3  "opmode_1_rst_out1"
  opmode_0_rst/1 -> Mux/3  "opmode_0_rst_out1"
  cram/1(Out) -> Reinterpret2/1  "cram_out1"
  Register/1 -> cram/2(In2)  "Register_out1"
  DSP48E_1/1 -> cram/1(In1)  "DSP48E_1_out1"
  Slice/1 -> Reinterpret/1  "Slice_out1"
  Reinterpret2/1 -> +=b/1
  Convert/1 -> Reinterpret1/1  "Convert_out1"
  Reinterpret/1 -> DSP48E_0/3  "Reinterpret_out1"
  DSP48E_0/1 -> Register/1  "DSP48E_0_out1"
  Mux1/1 -> Delay1/1  "Mux1_out1"
  Mux/1 -> DSP48E_0/4  "Mux_out1"
  Delay1/1 -> DSP48E_1/3  "Delay1_out1"
  DSP48_AB_splitter1/2(B) -> DSP48E_0/2  "DSP48_AB_splitter1_out2"
  DSP48_AB_splitter1/1(A) -> DSP48E_0/1  "DSP48_AB_splitter1_out1"
  DSP48E_0/2 -> DSP48E_1/5  "DSP48E_0_out2"
  b/1 -> Convert/1

== system kurtosis/kurtosis/kurtosis_acc_bank_8/abs_x_sq_acc ==
  sync : Inport
  b : Inport  Port=2
  Convert : xbsIndex_r4/Convert  gui_display_data_type=Fixed-point  arith_type="Signed  (2's comp)"  n_bits=96  bin_pt=34  float_type=Single  exp_bits=8  fraction_bits=24  quantization=Truncate  overflow=Wrap  en=off  latency=0  dbl_ovrd=off  pipeline=off  block_type=convert
  DSP48E_0 : xbsIndex_r4/DSP48E  use_a=Direct from A Port  use_b=Direct from B Port  reset_preg=off  pattern_from_creg=on  pattern='000000000000'  mask_from_creg=on  pattern_mask='000000000000'  sel_rounding_mask=Select mask  use_op=off  use_creg=on  rst_all=off  en_all=off  use_pcin=off  use_carrycascin=off  use_multsignin=off  use_carryout=on  use_patterndetect=off  use_patternbdetect=off  use_overflow=off  use_underflow=off  use_acout=off  use_bcout=off  use_pcout=off  use_multsignout=off  use_carrycascout=off  pipeline_a=1  pipeline_b=1  pipeline_acout=1  pipeline_bcout=1  pipeline_c=on  pipeline_p=on  pipeline_mult=on  pipeline_opmode=on  pipeline_alumode=on  pipeline_carryin=on  pipeline_carryinsel=on  rst_a=off  rst_b=off  rst_c=off  rst_mult=off  rst_p=off  rst_carry_in=off  rst_alumode=off  rst_ctrl=off  en_a1=off  en_a2=off  en_b1=off  en_b2=off  en_c=off  en_mult=off  en_p=off  en_carry_in=off  en_alumode=off  en_multcarryin=off  en_ctrl=off  use_synth_model=off  addsub_mode=ONE48  xl_useadderonly=off  block_type=dsp48e
  DSP48E_1 : xbsIndex_r4/DSP48E  use_a=Direct from A Port  use_b=Direct from B Port  reset_preg=off  pattern_from_creg=on  pattern='000000000000'  mask_from_creg=on  pattern_mask='000000000000'  sel_rounding_mask=Select mask  use_op=off  use_creg=off  rst_all=off  en_all=off  use_pcin=off  use_carrycascin=off  use_multsignin=off  use_carryout=off  use_patterndetect=off  use_patternbdetect=off  use_overflow=off  use_underflow=off  use_acout=off  use_bcout=off  use_pcout=off  use_multsignout=off  use_carrycascout=off  pipeline_a=2  pipeline_b=2  pipeline_acout=1  pipeline_bcout=1  pipeline_c=on  pipeline_p=on  pipeline_mult=on  pipeline_opmode=on  pipeline_alumode=on  pipeline_carryin=off  pipeline_carryinsel=on  rst_a=off  rst_b=off  rst_c=off  rst_mult=off  rst_p=off  rst_carry_in=off  rst_alumode=off  rst_ctrl=off  en_a1=off  en_a2=off  en_b1=off  en_b2=off  en_c=off  en_mult=off  en_p=off  en_carry_in=off  en_alumode=off  en_multcarryin=off  en_ctrl=off  use_synth_model=off  addsub_mode=ONE48  xl_useadderonly=off  block_type=dsp48e
  DSP48_AB_splitter1 : Subsystem
  DSP48_AB_splitter2_sub : Subsystem
  Delay1 : xbsIndex_r4/Delay  rst=off  infoeditControl=Selection of Reset will increase slice count due to use of real FFs and instead of SRLs  en=off  latency=1  dbl_ovrd=off  reg_retiming=off  block_type=delay
  Mux : xbsIndex_r4/Mux  inputs=2  en=off  latency=0  precision=Full  arith_type=Unsigned  n_bits=16  bin_pt=14  quantization=Truncate  overflow=Wrap  dbl_ovrd=off  block_type=mux
  Mux1 : xbsIndex_r4/Mux  inputs=2  en=off  latency=0  precision=Full  arith_type=Unsigned  n_bits=16  bin_pt=14  quantization=Truncate  overflow=Wrap  dbl_ovrd=off  block_type=mux
  Register : xbsIndex_r4/Register  init=0  rst=off  en=off  dbl_ovrd=off  block_type=register
  Reinterpret : xbsIndex_r4/Reinterpret  force_arith_type=on  arith_type="Signed  (2's comp)"  force_bin_pt=on  bin_pt=0  block_type=reinterpret
  Reinterpret1 : xbsIndex_r4/Reinterpret  force_arith_type=on  arith_type="Signed  (2's comp)"  force_bin_pt=on  bin_pt=0  block_type=reinterpret
  Reinterpret2 : xbsIndex_r4/Reinterpret  force_arith_type=on  arith_type="Signed  (2's comp)"  force_bin_pt=on  bin_pt=34  block_type=reinterpret
  Slice : xbsIndex_r4/Slice  nbits=48  boolean_output=off  mode=Lower Bit Location + Width  bit1=0  base1=MSB of Input  bit0=0  base0=LSB of Input  dbl_ovrd=off  block_type=slice
  Slice2 : xbsIndex_r4/Slice  nbits=48  boolean_output=off  mode=Lower Bit Location + Width  bit1=0  base1=MSB of Input  bit0=48  base0=LSB of Input  dbl_ovrd=off  block_type=slice
  cram : Subsystem
  dsp48e_ctrl_init_xblock124 : Subsystem
  dsp48e_ctrl_init_xblock125 : Subsystem
  opmode_0_rst : xbsIndex_r4/Constant  const=12  gui_display_data_type=Fixed-point  arith_type=Unsigned  n_bits=7  bin_pt=0  preci_type=Single  exp_width=8  frac_width=24  explicit_period=on  period=1  equ=P=C  opselect=C  inp2=PCIN>>17  opr=+  inp1=P  carry=CIN  dbl_ovrd=off  block_type=constant
  opmode_1_rst : xbsIndex_r4/Constant  const=3  gui_display_data_type=Fixed-point  arith_type=Unsigned  n_bits=7  bin_pt=0  preci_type=Single  exp_width=8  frac_width=24  explicit_period=on  period=1  equ=P=C  opselect=C  inp2=PCIN>>17  opr=+  inp1=P  carry=CIN  dbl_ovrd=off  block_type=constant
  zero : xbsIndex_r4/Constant  const=0  gui_display_data_type=Fixed-point  arith_type=Signed (2's comp)  n_bits=48  bin_pt=0  preci_type=Single  exp_width=8  frac_width=24  explicit_period=on  period=1  equ=P=C  opselect=C  inp2=PCIN>>17  opr=+  inp1=P  carry=CIN  dbl_ovrd=off  block_type=constant
  +=b : Outport
  wires:
  sync/1 -> Mux1/1, Mux/1
  Reinterpret1/1 -> Slice2/1, Slice/1  "Reinterpret1_out1"
  dsp48e_ctrl_init_xblock125/4(carryinsel) -> DSP48E_1/6  "dsp48e_ctrl1_out4"
  dsp48e_ctrl_init_xblock125/2(alumode) -> DSP48E_1/4  "dsp48e_ctrl1_out2"
  dsp48e_ctrl_init_xblock125/1(opmode) -> Mux1/2  "dsp48e_ctrl1_out1"
  dsp48e_ctrl_init_xblock124/4(carryinsel) -> DSP48E_0/7  "dsp48e_ctrl0_out4"
  dsp48e_ctrl_init_xblock124/3(carryin) -> DSP48E_0/6  "dsp48e_ctrl0_out3"
  dsp48e_ctrl_init_xblock124/2(alumode) -> DSP48E_0/5  "dsp48e_ctrl0_out2"
  dsp48e_ctrl_init_xblock124/1(opmode) -> Mux/2  "dsp48e_ctrl0_out1"
  DSP48_AB_splitter2_sub/2(B) -> DSP48E_1/2  "DSP48_AB_splitter2_out2"
  DSP48_AB_splitter2_sub/1(A) -> DSP48E_1/1  "DSP48_AB_splitter2_out1"
  Slice2/1 -> DSP48_AB_splitter2_sub/1(A:B)  "Slice2_out1"
  zero/1 -> DSP48_AB_splitter1/1(A:B)  "zero_out1"
  opmode_1_rst/1 -> Mux1/3  "opmode_1_rst_out1"
  opmode_0_rst/1 -> Mux/3  "opmode_0_rst_out1"
  cram/1(Out) -> Reinterpret2/1  "cram_out1"
  Register/1 -> cram/2(In2)  "Register_out1"
  DSP48E_1/1 -> cram/1(In1)  "DSP48E_1_out1"
  Slice/1 -> Reinterpret/1  "Slice_out1"
  Reinterpret2/1 -> +=b/1
  Convert/1 -> Reinterpret1/1  "Convert_out1"
  Reinterpret/1 -> DSP48E_0/3  "Reinterpret_out1"
  DSP48E_0/1 -> Register/1  "DSP48E_0_out1"
  Mux1/1 -> Delay1/1  "Mux1_out1"
  Mux/1 -> DSP48E_0/4  "Mux_out1"
  Delay1/1 -> DSP48E_1/3  "Delay1_out1"
  DSP48_AB_splitter1/2(B) -> DSP48E_0/2  "DSP48_AB_splitter1_out2"
  DSP48_AB_splitter1/1(A) -> DSP48E_0/1  "DSP48_AB_splitter1_out1"
  DSP48E_0/2 -> DSP48E_1/5  "DSP48E_0_out2"
  b/1 -> Convert/1

== system kurtosis/kurtosis/kurtosis_acc_bank_8/acc_rst ==
  sync : Inport
  Constant5 : xbsIndex_r4/Constant  const=1023  gui_display_data_type=Fixed-point  arith_type=Unsigned  n_bits=11  bin_pt=0  preci_type=Single  exp_width=8  frac_width=24  explicit_period=on  period=1  equ=P=C  opselect=C  inp2=PCIN>>17  opr=+  inp1=P  carry=CIN  dbl_ovrd=off  block_type=constant
  Counter : xbsIndex_r4/Counter  cnt_type=Free Running  cnt_to=Inf  operation=Up  start_count=0  cnt_by_val=1  arith_type=Unsigned  n_bits=10  bin_pt=0  load_pin=off  rst=on  en=off  explicit_period=on  period=1  dbl_ovrd=off  use_behavioral_HDL=off  implementation=Fabric  block_type=counter
  Logical : xbsIndex_r4/Logical  logical_function=OR  inputs=2  en=off  latency=0  precision=Full  arith_type=Unsigned  n_bits=16  bin_pt=0  align_bp=on  dbl_ovrd=off  block_type=logical
  Relational : xbsIndex_r4/Relational  mode=a=b  en=off  latency=0  dbl_ovrd=off  block_type=relational
  acc_del : xbsIndex_r4/Delay  rst=off  infoeditControl=Selection of Reset will increase slice count due to use of real FFs and instead of SRLs  en=off  latency=2  dbl_ovrd=off  reg_retiming=off  block_type=delay
  sync_del : xbsIndex_r4/Delay  rst=off  infoeditControl=Selection of Reset will increase slice count due to use of real FFs and instead of SRLs  en=off  latency=1  dbl_ovrd=off  reg_retiming=off  block_type=delay
  acc_rst : Outport
  sync_out : Outport  Port=2
  wires:
  sync/1 -> Logical/2, Counter/1
  Relational/1 -> sync_del/1, acc_del/1  "Relational_out1"
  sync_del/1 -> Logical/1  "sync_del_out1"
  acc_del/1 -> sync_out/1
  Constant5/1 -> Relational/2  "Constant5_out1"
  Counter/1 -> Relational/1  "Counter_out1"
  Logical/1 -> acc_rst/1

== system kurtosis/kurtosis/kurtosis_acc_bank_8/x_acc ==
  sync : Inport
  x : Inport  Port=2
  c_to_ri : Subsystem
  im_acc : Subsystem
  re_acc : Subsystem
  x_re_acc : Outport
  x_im_acc : Outport  Port=2
  wires:
  sync/1 -> im_acc/1(sync), re_acc/1(sync)
  im_acc/1(+=b) -> x_im_acc/1
  c_to_ri/2(im) -> im_acc/2(b)  "x_im"
  re_acc/1(+=b) -> x_re_acc/1
  c_to_ri/1(re) -> re_acc/2(b)  "x_re"
  x/1 -> c_to_ri/1(c)

== system kurtosis/kurtosis/kurtosis_acc_bank_8/x_cube_acc ==
  sync : Inport
  x : Inport  Port=2
  c_to_ri : Subsystem
  im_acc : Subsystem
  re_acc : Subsystem
  x_re_acc : Outport
  x_im_acc : Outport  Port=2
  wires:
  sync/1 -> im_acc/1(sync), re_acc/1(sync)
  im_acc/1(+=b) -> x_im_acc/1
  c_to_ri/2(im) -> im_acc/2(b)  "x_im"
  re_acc/1(+=b) -> x_re_acc/1
  c_to_ri/1(re) -> re_acc/2(b)  "x_re"
  x/1 -> c_to_ri/1(c)

== system kurtosis/kurtosis/kurtosis_acc_bank_8/x_sq_acc ==
  sync : Inport
  x : Inport  Port=2
  c_to_ri : Subsystem
  im_acc : Subsystem
  re_acc : Subsystem
  x_re_acc : Outport
  x_im_acc : Outport  Port=2
  wires:
  sync/1 -> im_acc/1(sync), re_acc/1(sync)
  im_acc/1(+=b) -> x_im_acc/1
  c_to_ri/2(im) -> im_acc/2(b)  "x_im"
  re_acc/1(+=b) -> x_re_acc/1
  c_to_ri/1(re) -> re_acc/2(b)  "x_re"
  x/1 -> c_to_ri/1(c)
